simulink model "torqueBalancingPHRIStandup_WBTv5"  (Simulink 9.1)
settings: Solver=FixedStepDiscrete  StartTime=0.0  StopTime="Config.SIMULATION_TIME "  FixedStep=Config.Ts  RelTol=1e-3  EnableMultiTasking=on
StopFcn:
  | cd(fileparts(which(bdroot)));
  | stopTorqueBalancingPHRIStandup;
undefined symbols (not defined in the file or in its folder): ASSISTANT_DOF_FOR_SIMULINK, bVectorConstraintsFeet, bVectorConstraintsLegs, Config, ConstraintsMatrixFeet, ConstraintsMatrixLegs, DiscIntNeverNeededParam, Gain, Reg, ROBOT_DOF, ROBOT_DOF_FOR_SIMULINK, Sat, Sm
libraries: WBToolboxLibrary x155, simulink x5
(part 4 of 4)

== matlab function Robot system/Robot State and References/Internal Coordinator/Compute State Velocity/Compute Base Velocity ==
  data: J_LeftFoot input double; J_RightFoot input double; feetInContact input double; nu_b output double; qjDot input double; Reg parameter double
function nu_b = computeBaseVelocityFCN(J_LeftFoot, J_RightFoot, feetInContact, qjDot, Reg)

    nu_b = computeBaseVelocity(J_LeftFoot, J_RightFoot, feetInContact, qjDot, Reg);
end

== matlab function Robot system/Dynamics and Kinematics/Dynamics/Add motors reflected inertias/Add motor reflected inertias ==
  data: M input double; M_with_inertia output double; Config parameter double
function M_with_inertia = addMotorsInertiaFCN(M,Config)

    M_with_inertia = addMotorsInertia(M,Config);

end

== matlab function Robot system/Robot State and References/State Machine Standup/Compute State Velocity/Compute Base Velocity ==
  data: J_LeftFixedLink input double; J_RightFixedLink input double; feetInContact input double; nu_b output double; qjDot input double; Reg parameter double
function nu_b = computeBaseVelocityFCN(J_LeftFixedLink, J_RightFixedLink, feetInContact, qjDot, Reg)

    nu_b = computeBaseVelocity(J_LeftFixedLink, J_RightFixedLink, feetInContact, qjDot, Reg);
end

== matlab function Robot system/Robot State and References/State Machine Standup/Compute base to fixed link transform/LFoot to base link transform /fromImuToHomogeousTransformFCN ==
  data: imu_H_link input double; imu_H_link_0 input double; link_H_base input double; inertial_0 input double; inertial input double; neck_pos input double; w_H_b output double; Config parameter double
function w_H_b = worldToBaseTransformWithIMUFCN(imu_H_link,imu_H_link_0,link_H_base,inertial_0,inertial,neck_pos,Config)

    w_H_b = worldToBaseTransformWithIMU(imu_H_link,imu_H_link_0,link_H_base,inertial_0,inertial,neck_pos,Config);

end

== matlab function Robot system/Dynamics and Kinematics/Kinematics/Legs in Contact ==
  data: icubStandup input double; legsInContact output double; state input double
function legsInContact = legsContactDetectorFCN(icubStandup,state)

   legsInContact = legsContactDetector(icubStandup,state);
end

== matlab function Robot system/Robot State and References/Internal Coordinator/Reference Generator CoM ==
  data: pos_CoM_0 input double; t input double; references_CoM output double; Config parameter double
function references_CoM = referenceGeneratorCoMFCN(pos_CoM_0, t, Config)

    references_CoM = referenceGeneratorCoM(pos_CoM_0, t, Config);
end

== matlab function Robot system/controller_QP/Compute angular momentum integral/Legs in Contact ==
  data: icubStandup input double; legsInContact output double; state input double
function legsInContact = legsContactDetectorFCN(icubStandup,state)

   legsInContact = legsContactDetector(icubStandup,state);
end

== matlab function Robot system/controller_QP/Compute joint torques (motor reflected inertia)/(transpose(T*Gamma))^{-1}*I_m*(T*Gamma)^{-1} ==
  data: reflectedInertia output double; Config parameter double
function reflectedInertia  = computeMotorsInertiaFCN(Config)

    [reflectedInertia] = computeMotorsInertia(Config);

end

== matlab function Robot system/Robot State and References/State Machine Standup/stateMachineStandupFCN ==
  data: wrench_rightFoot input double; wrench_leftFoot input double; w_H_b output double; constraints output double; CoM_des output double; qj_des output double; wrench_leftHand input double; wrench_rightHand input double; xCoM_0 input double; qj_0 input double; xCoM input double; l_sole_H_b input double; l_upper_leg_contact_H_b input double; t input double; STANDUP_WITH_ASSISTANT_FORCE input double; MEASURED_FT input double; STANDUP_WITH_ASSISTANT_TORQUE input double; Sm parameter double; impedances output double; KPCoM output double; KDCoM output double; Gain parameter double; currentState output double; jointsAndCoMSmoothingTime output double; fArms_phri input double
function [w_H_b, constraints, CoM_des, qj_des, impedances, KPCoM, KDCoM, currentState, jointsAndCoMSmoothingTime] = ...
             stateMachineStandupFCN(wrench_rightFoot, wrench_leftFoot, wrench_leftHand, wrench_rightHand, xCoM_0, qj_0, xCoM, l_sole_H_b, l_upper_leg_contact_H_b, t, STANDUP_WITH_ASSISTANT_FORCE, MEASURED_FT, STANDUP_WITH_ASSISTANT_TORQUE, Sm, Gain, fArms_phri)
         
         [w_H_b, constraints, CoM_des, qj_des, impedances, KPCoM, KDCoM, currentState, jointsAndCoMSmoothingTime] = ...
             stateMachineStandup(wrench_rightFoot, wrench_leftFoot, wrench_leftHand, wrench_rightHand, xCoM_0, qj_0, xCoM, l_sole_H_b, l_upper_leg_contact_H_b, t, STANDUP_WITH_ASSISTANT_FORCE, MEASURED_FT, STANDUP_WITH_ASSISTANT_TORQUE, Sm, Gain, fArms_phri);
end

== matlab function Robot system/Robot State and References/State Machine Standup/Compute State Velocity/Fixed Links Jacobians/Legs in Contact ==
  data: icubStandup input double; legsInContact output double; state input double
function legsInContact = legsContactDetectorFCN(icubStandup,state)

   legsInContact = legsContactDetector(icubStandup,state);
end

== matlab function Robot system/robot world to assistant feet transformation/MATLAB Function ==
  data: w_H_humanLeftFeet output double; w_H_robotLeftFeet input double; w_H_robotRightFeet input double; w_H_humanRightFeet output double
function [w_H_humanLeftFeet, w_H_humanRightFeet ]= fcn(w_H_robotLeftFeet,w_H_robotRightFeet)

    %% Fixed transformation from the robot feet to human feet defined
    %  human-forces-provider module configuration
    robotLeftFeet_H_humanLeftFeet = [-1.0   0.0     0.0     0.59;
                                      0.0  -1.0     0.0    -0.2549;
                                      0.0   0.0     1.0     0.0;
                                      0.0   0.0     0.0     1.0];
                                  
    robotRightFeet_H_humanRightFeet = [-1.0   0.0     0.0     0.59;
                                        0.0  -1.0     0.0    -0.2549;
                                        0.0   0.0     1.0     0.0;
                                        0.0   0.0     0.0     1.0];
                                  
    w_H_humanLeftFeet  = w_H_robotLeftFeet * robotLeftFeet_H_humanLeftFeet;
    
    w_H_humanRightFeet = w_H_robotRightFeet * robotRightFeet_H_humanRightFeet;

end

== matlab function Assistant system/Real system/Robot Assistant Position Control/getJointRef ==
  data: sim_time input double; q input double; state input double; joint_ref output double
function joint_ref = getJointRef(sim_time, q, state)

    joint_ref        = q;
                        % Torso                       % Left arm                               % Right arm                             % Left leg                                                 % Right leg   
    joint_references = [-0.0000   -0.0000   -0.0000   0.1050    0.3630    0.0785    0.9367    -0.0349    0.3053    0.2791    0.9856    0.0000    0.0000   -0.0000   -0.0000   -0.0000  -0.0000    0.0000    0.0000   -0.0000   -0.0000   -0.0000  -0.0000;
                        -0.0000   -0.0000   -0.0000  -0.1660    0.4466    0.1954    0.5862    -0.1082    0.5582    0.4120    0.7940    0.0000    0.0000   -0.0000   -0.0000   -0.0000  -0.0000    0.0000    0.0000   -0.0000   -0.0000   -0.0000  -0.0000;
                        -0.0000   -0.0000   -0.0000  -0.1832    0.2800    0.0611    1.4500    -0.1832    0.2800    0.0611    1.4500    0.0000    0.0000   -0.0000   -0.0000   -0.0000  -0.0000    0.0000    0.0000   -0.0000   -0.0000   -0.0000  -0.0000];

% %                     joint_references = [-0.0000   -0.0000   -0.0000   0.1050    0.3630    0.0785    0.9367    -0.0349    0.3053    0.2791    0.9856    0.2130    0.0890   -0.0000   -0.1750   -0.0733  -0.0907    0.2130    0.0890   -0.0000   -0.1750   -0.0733  -0.0907;
% %                         -0.0000   -0.0000   -0.0000  -0.1660    0.4466    0.1954    0.5862    -0.1082    0.5582    0.4120    0.7940    0.2130    0.0890   -0.0000   -0.1750   -0.0733  -0.0907    0.2130    0.0890   -0.0000   -0.1750   -0.0733  -0.0907;
% %                         -0.0000   -0.0000   -0.0000  -0.1660    0.4466    0.1954    0.5862    -0.1082    0.5582    0.4120    0.7940    0.2130    0.0890   -0.0000   -0.1750   -0.0733  -0.0907    0.2130    0.0890   -0.0000   -0.1750   -0.0733  -0.0907;
% %                         -0.0000   -0.0000   -0.0000  -0.1660    0.4466    0.1954    0.5862    -0.1082    0.5582    0.4120    0.7940    0.2130    0.0890   -0.0000   -0.1750   -0.0733  -0.0907    0.2130    0.0890   -0.0000   -0.1750   -0.0733  -0.0907];
% % -0.1832    0.2800    0.0611    1.4500    -0.1450    0.2512    0.1400    1.5100
% %     joint_ref    = joint_references(state,:)';
    
    if state < 4 && sim_time > 2
% %     if sim_time > 2

        joint_ref    = joint_references(state,:)';
        
    elseif state >= 4
        
        joint_ref    = joint_references(3,:)';
        
    end
              
end

== matlab function Robot system/controller_QP/Balancing Controller  ==
  data: tauModel output double; Sigma output double; NA output double; f_HDot output double; HessianMatrixQP1Foot output double; gradientQP1Foot output double; ConstraintsMatrixQP1Foot output double; bVectorConstraintsQp1Foot output double; HessianMatrixQP2FeetOrLegs output double; gradientQP2FeetOrLegs output double; ConstraintsMatrixQP2FeetOrLegs output double; bVectorConstraintsQp2FeetOrLegs output double; constraints input double; ROBOT_DOF_FOR_SIMULINK input double; ASSISTANT_DOF_FOR_SIMULINK input double; ConstraintsMatrix input double; bVectorConstraints input double; qj input double; qjDes input double; nu input double; M input double; h input double; L input double; intLw input double; w_H_l_contact input double; w_H_r_contact input double; JL input double; JR input double; dJL_nu input double; dJR_nu input double; xCoM input double; J_CoM input double; JDot_nu_CoM input double; desired_x_dx_ddx_CoM input double; CMM input double; gainsPCOM input double; gainsDCOM input double; impedances input double; Reg parameter double; errorCoM output double; f_noQP output double; Gain parameter double; w_H_lArm input double; w_H_rArm input double; JLArm input double; JRArm input double; dJLArm_nu input double; dJRArm_nu input double; LArmWrench input double; RArmWrench input double; STANDUP_WITH_ASSISTANT_FORCE input double; MEASURED_FT input double; STANDUP_WITH_ASSISTANT_TORQUE input double; TRAJECTORY_PARAMETRIZATION input double; assistant_w_H_b input double; assistant_qj input double; assistant_nu_b input double; assistant_dqj input double; assistant_M input double; assistant_h input double; assistant_torques input double; assistant_w_H_l_contact input double; assistant_w_H_r_contact input double; assistant_JL input double; assistant_JR input double; assistant_dJL_nu input double; assistant_dJR_nu input double; assistant_w_H_lArm_contact input double; assistant_w_H_rArm_contact input double; assistant_JLArm input double; assistant_JRArm input double; assistant_dJLArm_nu input double; assistant_dJRArm_nu input double; correctionFromSupportForce output double; L_error output double; V output double; alpha output double; state input double; robot_torques input double; fArms output double; phri_assistant_feet_wrench output double; phri_robot_feet_wrench output double; correctionFromSupportTorque output double; SOLO_ROBOT input double; sdot output double; SDOT_REG input double
function [tauModel, Sigma, NA, f_HDot, ...
          HessianMatrixQP1Foot, gradientQP1Foot, ConstraintsMatrixQP1Foot, bVectorConstraintsQp1Foot, ...
          HessianMatrixQP2FeetOrLegs, gradientQP2FeetOrLegs, ConstraintsMatrixQP2FeetOrLegs, bVectorConstraintsQp2FeetOrLegs, ...
          errorCoM, f_noQP, correctionFromSupportForce, L_error, V, alpha, fArms, phri_assistant_feet_wrench, phri_robot_feet_wrench, correctionFromSupportTorque, sdot] =  ...
              balancingControllerStandupFCN(constraints, ROBOT_DOF_FOR_SIMULINK, ASSISTANT_DOF_FOR_SIMULINK, ConstraintsMatrix, bVectorConstraints, ...
                                         qj, qjDes, nu, M, h, L, intLw, w_H_l_contact, w_H_r_contact, JL, JR, dJL_nu, dJR_nu, xCoM, J_CoM, JDot_nu_CoM, desired_x_dx_ddx_CoM, CMM, ...
                                         gainsPCOM, gainsDCOM, impedances, Reg, Gain, w_H_lArm, w_H_rArm, JLArm, JRArm, dJLArm_nu, dJRArm_nu,...
                                         LArmWrench, RArmWrench, STANDUP_WITH_ASSISTANT_FORCE, MEASURED_FT, STANDUP_WITH_ASSISTANT_TORQUE, TRAJECTORY_PARAMETRIZATION, ...
                                         assistant_w_H_b, assistant_qj, assistant_nu_b, assistant_dqj, assistant_M, assistant_h, assistant_torques, ...
                                         assistant_w_H_l_contact, assistant_w_H_r_contact, assistant_JL, assistant_JR, assistant_dJL_nu, assistant_dJR_nu,...
                                         assistant_w_H_lArm_contact, assistant_w_H_rArm_contact, assistant_JLArm, assistant_JRArm, assistant_dJLArm_nu, assistant_dJRArm_nu,...
                                         state, robot_torques, SOLO_ROBOT, SDOT_REG)
           
   [tauModel, Sigma, NA, f_HDot, ...
          HessianMatrixQP1Foot, gradientQP1Foot, ConstraintsMatrixQP1Foot, bVectorConstraintsQp1Foot, ...
          HessianMatrixQP2FeetOrLegs, gradientQP2FeetOrLegs, ConstraintsMatrixQP2FeetOrLegs, bVectorConstraintsQp2FeetOrLegs, ...
          errorCoM, f_noQP, correctionFromSupportForce, L_error, V, alpha, fArms, phri_assistant_feet_wrench, phri_robot_feet_wrench, correctionFromSupportTorque, sdot] =  ...
              balancingControllerStandup(constraints, ROBOT_DOF_FOR_SIMULINK, ASSISTANT_DOF_FOR_SIMULINK, ConstraintsMatrix, bVectorConstraints, ...
                                         qj, qjDes, nu, M, h, L, intLw, w_H_l_contact, w_H_r_contact, JL, JR, dJL_nu, dJR_nu, xCoM, J_CoM, JDot_nu_CoM, desired_x_dx_ddx_CoM, CMM, ...
                                         gainsPCOM, gainsDCOM, impedances, Reg, Gain, w_H_lArm, w_H_rArm, JLArm, JRArm, dJLArm_nu, dJRArm_nu,...
                                         LArmWrench, RArmWrench, STANDUP_WITH_ASSISTANT_FORCE, MEASURED_FT, STANDUP_WITH_ASSISTANT_TORQUE, TRAJECTORY_PARAMETRIZATION, ...
                                         assistant_w_H_b, assistant_qj, assistant_nu_b, assistant_dqj, assistant_M, assistant_h, assistant_torques, ...
                                         assistant_w_H_l_contact, assistant_w_H_r_contact, assistant_JL, assistant_JR, assistant_dJL_nu, assistant_dJR_nu,...
                                         assistant_w_H_lArm_contact, assistant_w_H_rArm_contact, assistant_JLArm, assistant_JRArm, assistant_dJLArm_nu, assistant_dJRArm_nu,...
                                         state, robot_torques, SOLO_ROBOT, SDOT_REG);
end

== matlab function Robot system/emergency stop: joint limits/MATLAB Function ==
  data: umin input double; umax input double; u input double; inRange output double; tol input double
function inRange = checkRangeFCN(umin, umax, u, tol)

    inRange = checkRange(umin, umax, u, tol);
end

== matlab function Robot system/Robot State and References/Select State and References/Analytical Min-jerk Trajectory ==
  data: xCoM_0 input double; CoMDes input double; position output double; period input double; t input double; tBalancing input double; state input double; velocity output double; acceleration output double; s input double; sdot input double; sdotdot input double; trajectory_parametrization input double
function [position, velocity, acceleration] = fcn(xCoM_0, CoMDes, period, t, tBalancing, state, s, sdot, sdotdot, trajectory_parametrization)

    persistent CoM_initial;
    persistent CoM_final;
    persistent elapsedTime;
    persistent durationVector;
    persistent duration;
    persistent updateFlag;
    persistent sdotvalue;
    persistent sdotdotvalue;
    persistent svalue;
    persistent stopstate;
    
    if isempty(CoM_initial) || isempty(CoM_final) || isempty(elapsedTime) || isempty(durationVector) || isempty(duration) ||...
       isempty(updateFlag) || isempty(svalue) || isempty(sdotvalue) || isempty(sdotdotvalue) || isempty(stopstate)
        
        CoM_initial        = xCoM_0;
        CoM_final          = xCoM_0;
        elapsedTime        = 0;
        durationVector     = [tBalancing, 1.5, 0.5, 1.8];
        duration           = durationVector(1);
        updateFlag         = false;
        
        svalue             = t;
        sdotvalue          = 1; %% default values
        sdotdotvalue       = 1;
        
        stopstate          = 4;
        
    end
    
    %% MOVE COM FORWARD
    if state == 2
        
        if (~updateFlag)
            
            elapsedTime = elapsedTime + durationVector(state-1) ;
            
            duration = durationVector(state);
        
            CoM_initial = CoM_final;
            CoM_final   = CoMDes(1:3);
            
            updateFlag = true;
            
        end
        
    end
    
    %% TWO FEET BALANCING
    if state == 3
        
        if (updateFlag)
            
            elapsedTime = elapsedTime + durationVector(state-1);
            
            duration = durationVector(state);

            CoM_initial = CoM_final;
            CoM_final   = CoMDes(1:3);
            
            updateFlag = false;
            
        end
        
    end
    
    %% LIFTING UP
    if state == 4
        
        if (~updateFlag)
            
            elapsedTime = elapsedTime + durationVector(state-1);
            
            duration = durationVector(state);

            CoM_initial = CoM_final;
            CoM_final   = CoMDes(1:3);
            
            updateFlag = true;
            
        end
        
    end
    
    %% Use the feedback terms
    if (trajectory_parametrization)
        svalue = s; %% new parametrization
        sdotvalue = sdot; 
        sdotdotvalue = sdotdot;
    else
        svalue = t; %% time parametrization
    end
    
    %% free parameter
    time = svalue - elapsedTime - period;
    
    %% Final standing stage
    if ((state == stopstate) && (elapsedTime + time >= sum(durationVector(1:stopstate))))
        
        if (updateFlag)
            
            CoM_initial = CoM_final;
            
            updateFlag = false;
            
        end
        
    end

    %% Compute min-jerk trajectory
    a = (CoM_final - CoM_initial);
    b = (10 * (time/duration).^3 - 15 * (time/duration).^4 + 6 * (time/duration).^5)';

    %% Position
    position = CoM_initial + a * b;

    %% Velocity
    velocity = a.*(30 * (time/duration).^2 - 60 * (time/duration).^3 + 30 * (time/duration).^4)';

    %% Acceleration
    acceleration = a.*(60*(time/duration).^1 - 180*(time/duration).^2 + 120*(time/duration).^3)';
    
end

== matlab function Robot system/controller_QP/Compute angular momentum integral/References for H ==
  data: qjErr input double; JL input double; JR input double; nu_b_equivalent output double; Reg parameter double; activeFeetConstraints input double
function nu_b_equivalent = generateReferencesForH_FCN(qjErr, JL, JR, Reg, activeFeetConstraints)

    if activeFeetConstraints(1) == 1
    
        pinvJb          = (JL(:,1:6)'*JL(:,1:6) + Reg.pinvDamp_nu_b*eye(6))\JL(:,1:6)';
        nu_b_equivalent = -pinvJb*JL(:,7:end)*qjErr;
    else
    
        pinvJb          = (JR(:,1:6)'*JR(:,1:6) + Reg.pinvDamp_nu_b*eye(6))\JR(:,1:6)';
        nu_b_equivalent = -pinvJb*JR(:,7:end)*qjErr;
    end
end

== matlab function Robot system/Robot State and References/State Machine Standup/Visualise extrnal wrenches/Compute current threshold ==
  data: thresholdContactLeftHand output double; thresholdContactRightHand output double; state input double; thresholdContactLeftFoot output double; thresholdContactRightFoot output double; Sm parameter double
function [thresholdContactLeftHand,thresholdContactRightHand, ...
          thresholdContactLeftFoot,thresholdContactRightFoot] = currentThreshold(state,Sm)

    thresholdContactLeftHand  = Sm.wrench_thresholdContactLHand(state);
    thresholdContactRightHand = Sm.wrench_thresholdContactRHand(state);
    thresholdContactLeftFoot  = Sm.wrench_thresholdContactLFoot(state);
    thresholdContactRightFoot = Sm.wrench_thresholdContactRFoot(state);
end
